simulink model "direct_event1_eg_3"  (R2018a)
settings: Solver=VariableStepAuto  StartTime=0.0  StopTime=10.0  RelTol=1e-3
settings Model: Creator=86188  LastModifiedBy=86188

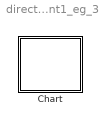
== system direct_event1_eg_3 ==
  Chart : Stateflow chart  TreatAsAtomicUnit=on

== stateflow chart direct_event1_eg_3/Chart ==
  state AM
    state A [parallel]
      settings: executionOrder=1
      state A2
      state A1
      (default) -> A1
      A1 -> A2 : [data==1]{send(E_one,B.B1.B2)}
      A2 -> A1 : E_two
    state B [parallel]
      settings: executionOrder=2
      state B1
        state B2
          state B21
          state B22
          (default) -> B21
          B21 -> B22 : E_one
        state B3
        (default) -> B2
        B2 -> B3 : E_two
        B3 -> B2 : E_one
      state B4
      (default) -> B1
      B1 -> B4 : E_one
      B4 -> B1 : E_two
  (default) -> AM
  data: data local =1
  events: E_one local FUNCTION_CALL_EVENT; E_two local FUNCTION_CALL_EVENT
